simulink model "plc"  (R2024b)
settings: Solver=VariableStepAuto  StartTime=0.0  StopTime=inf  RelTol=1e-3
values from neighbouring files (symbols this model uses):
  a1 = 0.45    [init.m]
  A1 = 100    [init.m]
  a2 = 0.25    [init.m]
  A2 = 100    [init.m]
  A3 = 100    [init.m]
  g = 980.665    [init.m]
  Q1_max = 100    [init.m]
  Q3_max = 100    [init.m]
  s12 = 0.5    [init.m]
  s23 = 0.5    [init.m]
libraries: dspnetwork x6
settings Model: Creator=Dottorandi  LastModifiedBy=mattia
settings SolverCC: AlgebraicLoopSolver=TrustRegion
settings DataIOCC: ReturnWorkspaceOutputs=off
settings DebuggingCC: UnconnectedInputMsg=warning  UnconnectedOutputMsg=warning  UnconnectedLineMsg=warning  ArithmeticOperatorsInVariantConditions=warning
settings ModelReferenceCC: EnableRefExpFcnMdlSchedulingChecks=on
settings SFSimCC: SimUseLocalCustomCode=off  CustomCodeUndefinedFunction=UseInterfaceOnly
settings RTWCC: RTWUseLocalCustomCode=off  GPUComputeCapability=3.5  DLArmComputeVersion=19.05

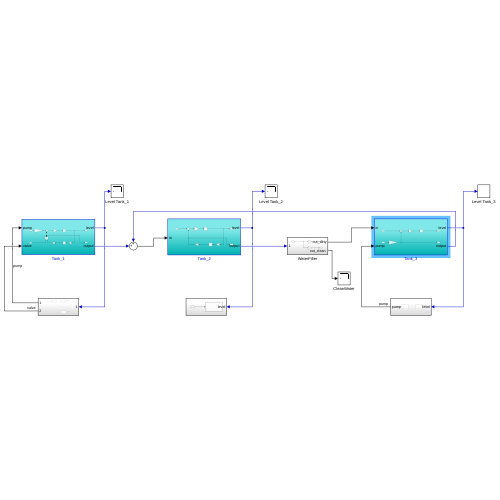
[thumbnail: Simulink's stored preview of the top-level diagram]
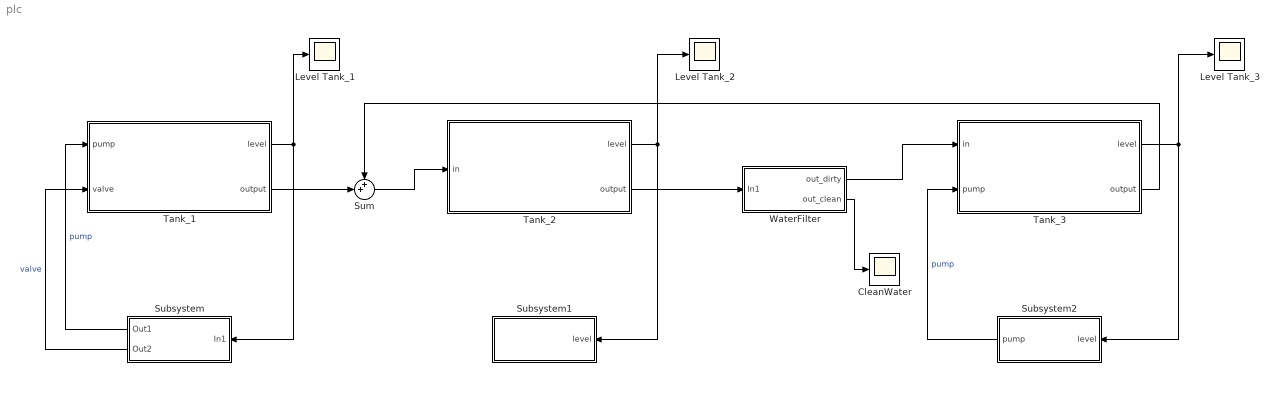
== system plc ==
  "CleanWater " : Scope
  Level Tank_1 : Scope
  Level Tank_2 : Scope
  Level Tank_3 : Scope
  Subsystem : Subsystem
  Subsystem1 : Subsystem
  Subsystem2 : Subsystem
  Sum : Sum  Inputs=++|
  Tank_1 : Subsystem
  Tank_2 : Subsystem
  Tank_3 : Subsystem
  WaterFilter : Subsystem
  wires:
  Sum/1 -> Tank_2/1(in)
  Tank_1/1(level) -> Level Tank_1/1, Subsystem/1(In1)
  Tank_3/2(output) -> Sum/1
  WaterFilter/2("out_clean ") -> "CleanWater "/1
  Tank_1/2(output) -> Sum/2
  Subsystem/2(Out2) -> Tank_1/2(valve)  "valve"
  Tank_2/2(output) -> WaterFilter/1(In1)
  Subsystem/1(Out1) -> Tank_1/1(pump)  "pump"
  WaterFilter/1(out_dirty) -> Tank_3/1(in)
  Subsystem2/1(pump) -> Tank_3/2(pump)  "pump"
  Tank_3/1(level) -> Level Tank_3/1, Subsystem2/1(level)
  Tank_2/1(level) -> Level Tank_2/1, Subsystem1/1(level)

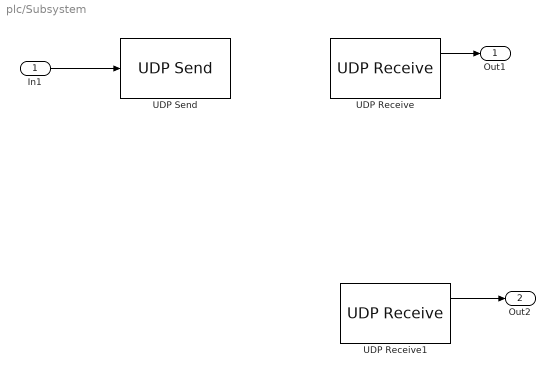
== system plc/Subsystem ==
  In1 : Inport
  UDP Receive : dspnetwork/UDP Receive  localURL='0.0.0.0'  localPort=10002  remoteURL='0.0.0.0'  remotePort=-1  recvBufferSize=2  dims=1  signalDatatype=uint16  isComplex=off  isVarSize=off  showBlockingTime=on  blockingTime=0  sampletime=1  blockPlatform=LINUX
  UDP Receive1 : dspnetwork/UDP Receive  localURL='0.0.0.0'  localPort=10003  remoteURL='0.0.0.0'  remotePort=-1  recvBufferSize=2  dims=1  signalDatatype=uint16  isComplex=off  isVarSize=off  showBlockingTime=on  blockingTime=0  sampletime=1  blockPlatform=LINUX
  UDP Send : dspnetwork/UDP Send  remoteURL='localhost'  remotePort=10001  localURL='255.255.255.255'  localPortSource=Automatically determine  localPort=-1  sendBufferSize=8192  sampletime=-1  blockPlatform=LINUX  separateLengthPort=0
  Out1 : Outport  VectorParamsAs1DForOutWhenUnconnected=off
  Out2 : Outport  Port=2  VectorParamsAs1DForOutWhenUnconnected=off
  wires:
  In1/1 -> UDP Send/1
  UDP Receive/1 -> Out1/1
  UDP Receive1/1 -> Out2/1

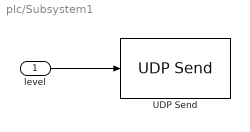
== system plc/Subsystem1 ==
  level : Inport
  UDP Send : dspnetwork/UDP Send  remoteURL='localhost'  remotePort=10004  localURL='255.255.255.255'  localPortSource=Automatically determine  localPort=-1  sendBufferSize=8192  sampletime=-1  blockPlatform=LINUX  separateLengthPort=0
  wires:
  level/1 -> UDP Send/1

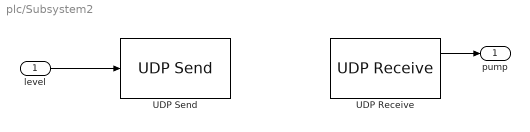
== system plc/Subsystem2 ==
  level : Inport
  UDP Receive : dspnetwork/UDP Receive  localURL='0.0.0.0'  localPort=10006  remoteURL='0.0.0.0'  remotePort=-1  recvBufferSize=2  dims=1  signalDatatype=uint16  isComplex=off  isVarSize=off  showBlockingTime=on  blockingTime=0  sampletime=1  blockPlatform=LINUX
  UDP Send : dspnetwork/UDP Send  remoteURL='localhost'  remotePort=10005  localURL='255.255.255.255'  localPortSource=Automatically determine  localPort=-1  sendBufferSize=8192  sampletime=-1  blockPlatform=LINUX  separateLengthPort=0
  pump : Outport  VectorParamsAs1DForOutWhenUnconnected=off
  wires:
  level/1 -> UDP Send/1
  UDP Receive/1 -> pump/1

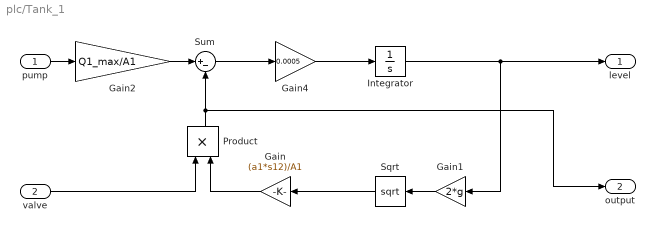
== system plc/Tank_1 ==
  pump : Inport
  valve : Inport  Port=2
  Gain : Gain  Gain=(a1*s12)/A1
  Gain1 : Gain  Gain=2*g
  Gain2 : Gain  Gain=Q1_max/A1
  Gain4 : Gain  Gain=0.0005
  Integrator : Integrator  InitialCondition=35  LimitOutput=on  UpperSaturationLimit=100  LowerSaturationLimit=0
  Product : Product
  Sqrt : Sqrt
  Sum : Sum  Inputs=|+-
  level : Outport  VectorParamsAs1DForOutWhenUnconnected=off
  output : Outport  Port=2  VectorParamsAs1DForOutWhenUnconnected=off
  wires:
  pump/1 -> Gain2/1
  Integrator/1 -> Gain1/1, level/1
  Gain/1 -> Product/2
  Sqrt/1 -> Gain/1
  Gain1/1 -> Sqrt/1
  valve/1 -> Product/1
  Product/1 -> Sum/2, output/1
  Gain2/1 -> Sum/1
  Sum/1 -> Gain4/1
  Gain4/1 -> Integrator/1

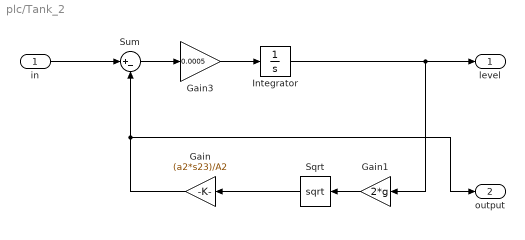
== system plc/Tank_2 ==
  in : Inport
  Gain : Gain  Gain=(a2*s23)/A2
  Gain1 : Gain  Gain=2*g
  Gain3 : Gain  Gain=0.0005
  Integrator : Integrator  LimitOutput=on  UpperSaturationLimit=30  LowerSaturationLimit=0
  Sqrt : Sqrt
  Sum : Sum  Inputs=|+-
  level : Outport  VectorParamsAs1DForOutWhenUnconnected=off
  output : Outport  Port=2  VectorParamsAs1DForOutWhenUnconnected=off
  wires:
  in/1 -> Sum/1
  Integrator/1 -> Gain1/1, level/1
  Sqrt/1 -> Gain/1
  Gain1/1 -> Sqrt/1
  Gain/1 -> output/1, Sum/2
  Sum/1 -> Gain3/1
  Gain3/1 -> Integrator/1

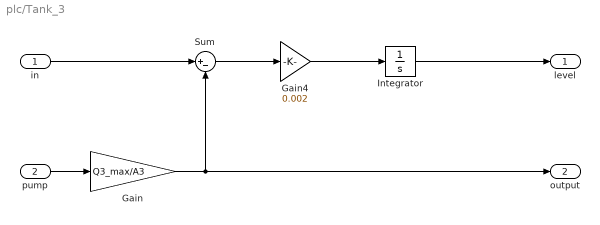
== system plc/Tank_3 ==
  in : Inport
  pump : Inport  Port=2
  Gain : Gain  Gain=Q3_max/A3
  Gain4 : Gain  Gain=0.002
  Integrator : Integrator  LimitOutput=on  UpperSaturationLimit=4  LowerSaturationLimit=0
  Sum : Sum  Inputs=|+-
  level : Outport  VectorParamsAs1DForOutWhenUnconnected=off
  output : Outport  Port=2  VectorParamsAs1DForOutWhenUnconnected=off
  wires:
  Integrator/1 -> level/1
  pump/1 -> Gain/1
  in/1 -> Sum/1
  Gain/1 -> Sum/2, output/1
  Sum/1 -> Gain4/1
  Gain4/1 -> Integrator/1

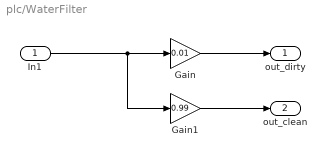
== system plc/WaterFilter ==
  In1 : Inport
  Gain : Gain  Gain=0.01
  Gain1 : Gain  Gain=0.99
  out_dirty : Outport  VectorParamsAs1DForOutWhenUnconnected=off
  "out_clean " : Outport  Port=2  VectorParamsAs1DForOutWhenUnconnected=off
  wires:
  In1/1 -> Gain1/1, Gain/1
  Gain/1 -> out_dirty/1
  Gain1/1 -> "out_clean "/1
